simulink model "MPC_mobile_base_ROS"  (R2018b)
settings: Solver=ode4  StartTime=0.0  StopTime=inf  FixedStep=T  RelTol=1e-3
values from neighbouring files (symbols this model uses):
  N = 3    [MPC_dyn_N=3arc traj.mat]    (also in MPC_dyn_N=3arc traj_active.mat; MPC_dyn_N=3complex traj.mat; MPC_dyn_N=3complex traj_active.mat; MPC_dyn_N=6arc traj.mat = 6)
  T = 0.5    [MPC_dyn_N=3arc traj.mat]    (also in MPC_dyn_N=3arc traj_active.mat; MPC_dyn_N=3complex traj.mat; MPC_dyn_N=3complex traj_active.mat; MPC_dyn_N=6arc traj.mat)
  xd = [0 0 0 0 0 0.000654498469498 0.0758636207458 4.96526307585e-05 0.00261799387799 0.227590374774 0.000446873251435 0.00589048622548 ... (153 elements, 3x51)]    [MPC_dyn_N=3arc traj.mat]    (also in MPC_dyn_N=3arc traj_active.mat; MPC_dyn_N=3complex traj.mat = [0 0 0 0.25 0 0 0.5 0 2.44929359829e-17 0.75 -0.024302237621; MPC_dyn_N=3complex traj_active.mat = [0 0 0 0.25 0 0 0.5 0 2.44929359829e-17 0.75 -0.024302237621; MPC_dyn_N=6arc traj.mat)
undefined symbols (not defined in the file or in its folder): Angular, Linear
libraries: simulink x6, robotlib x4, sharedtransform x1
settings Model: EnablePacing=on  Creator=RaffaelePC  LastModifiedBy=francesco
settings DebuggingCC: UnderSpecifiedDimensionMsg=warning

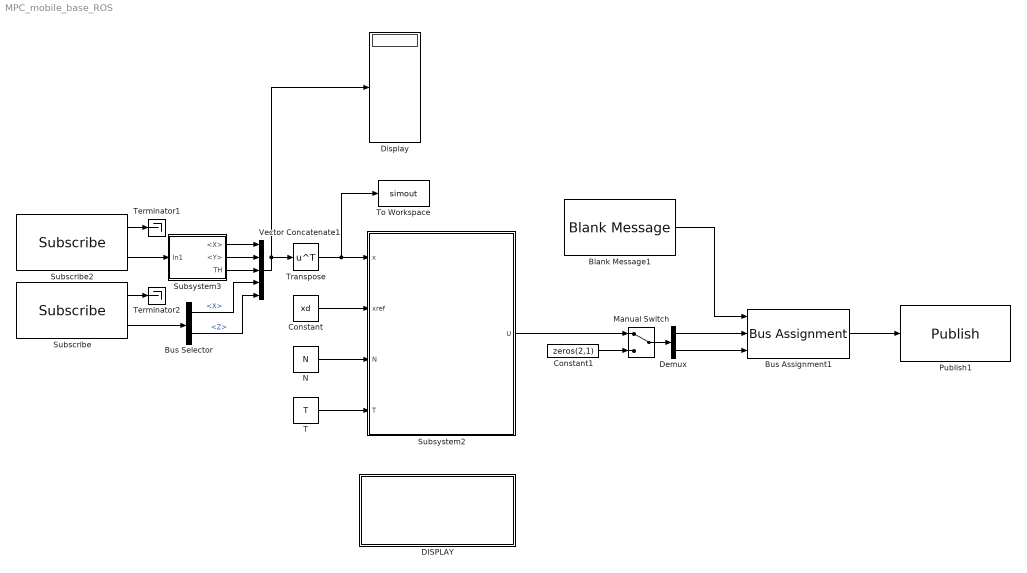
== system MPC_mobile_base_ROS ==
  Blank Message1 : robotlib/Blank Message  messageClass=Message  entityType=geometry_msgs/Twist  messageType=geometry_msgs/Twist  SampleTime=T
      settings: SourceProductBaseCode=RO
  Bus Assignment1 : BusAssignment  AssignedSignals=Linear.X,Angular.Z
  Bus Selector : BusSelector  OutputSignals=Linear.X,Angular.Z
  Constant : Constant  Value=xd
  Constant1 : Constant  Value=zeros(2,1)
  DISPLAY : Subsystem
  Demux : Demux  Outputs=2
  Display : Display
  Manual Switch : ManualSwitch
  N : Constant  Value=N
  Publish1 : robotlib/Publish  topicSource=Select from ROS network  topic=/cmd_vel  messageType=geometry_msgs/Twist  messageQueueLength=1
      settings: SourceProductBaseCode=RO
  Subscribe : robotlib/Subscribe  topicSource=Select from ROS network  topic=/cmd_vel  messageType=geometry_msgs/Twist  sampleTime=-1  messageQueueLength=1
      settings: SourceProductBaseCode=RO
  Subscribe2 : robotlib/Subscribe  topicSource=Select from ROS network  topic=/odom  messageType=nav_msgs/Odometry  sampleTime=T  messageQueueLength=1
      settings: SourceProductBaseCode=RO
  Subsystem2 : Subsystem
      mask Display: disp('MPC FINTO')
  Subsystem3 : Subsystem
  T : Constant  Value=T
  Terminator1 : Terminator
  Terminator2 : Terminator
  To Workspace : ToWorkspace  VariableName=simout  SaveFormat=Timeseries  SampleTime=-1
  Transpose : Math  Operator=transpose  SaturateOnIntegerOverflow=on
  Vector Concatenate1 : Concatenate  NumInputs=5
  wires:
  Demux/2 -> Bus Assignment1/3
  Manual Switch/1 -> Demux/1
  Constant1/1 -> Manual Switch/2
  Demux/1 -> Bus Assignment1/2
  Bus Assignment1/1 -> Publish1/1
  Blank Message1/1 -> Bus Assignment1/1
  Vector Concatenate1/1 -> Display/1, Transpose/1
  Transpose/1 -> To Workspace/1, Subsystem2/1(x)
  Constant/1 -> Subsystem2/2(xref)
  N/1 -> Subsystem2/3(N)
  T/1 -> Subsystem2/4(T)
  Subsystem2/1(U) -> Manual Switch/1
  Subsystem3/1(<X>) -> Vector Concatenate1/1
  Subsystem3/2(<Y>) -> Vector Concatenate1/2
  Subsystem3/3(TH) -> Vector Concatenate1/3
  Subscribe2/2 -> Subsystem3/1(In1)
  Subscribe2/1 -> Terminator1/1
  Subscribe/2 -> Bus Selector/1
  Bus Selector/1 -> Vector Concatenate1/4  "<X>"
  Bus Selector/2 -> Vector Concatenate1/5  "<Z>"
  Subscribe/1 -> Terminator2/1

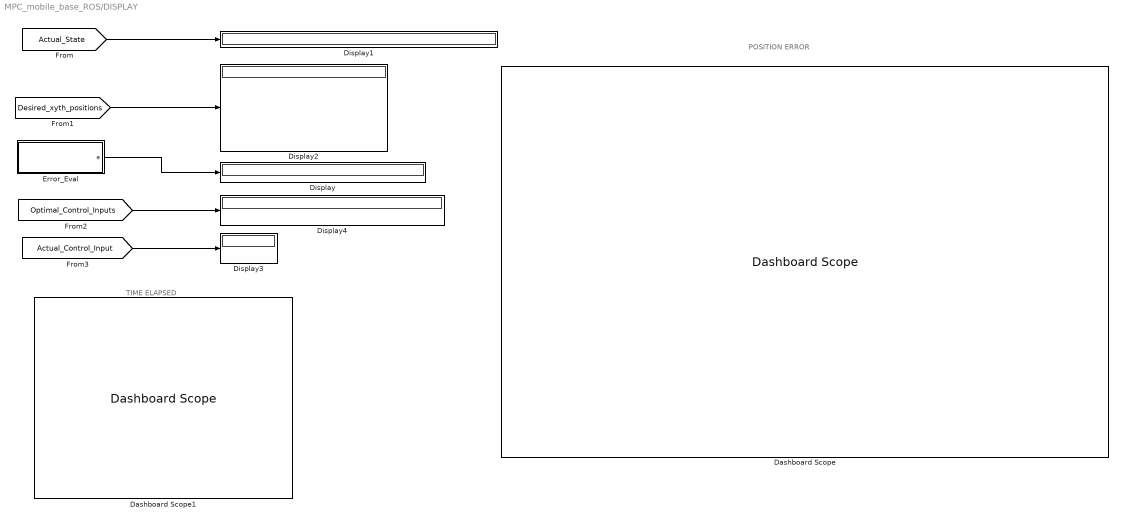
== system MPC_mobile_base_ROS/DISPLAY ==
  note: POSITION ERROR
  note: TIME ELAPSED
  Dashboard Scope : DashboardScope  WebBlockId=507  Ymin=-0.5  Ymax=0.5
  Dashboard Scope1 : DashboardScope  WebBlockId=516  Ymin=0  Ymax=1
  Display{,1..4} (5 alike) : Display
  "Error_Eval " : Subsystem
  wires:
  [Optimal_Control_Inputs] -> Display4/1
  [Desired_xyth_positions] -> Display2/1
  [Actual_Control_Input] -> Display3/1
  [Actual_State] -> Display1/1
  "Error_Eval "/1(e) -> Display/1

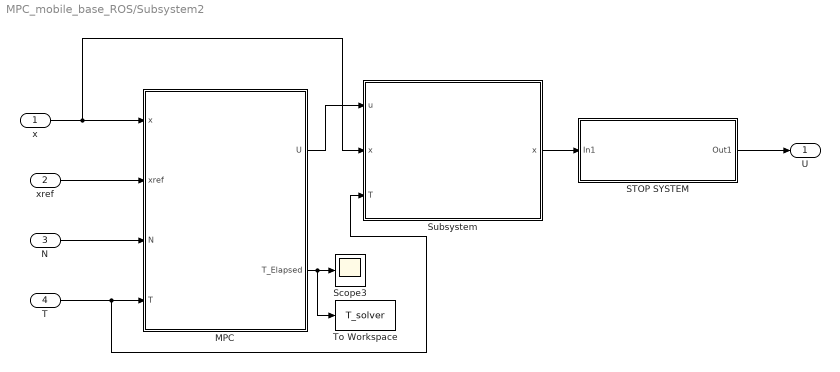
== system MPC_mobile_base_ROS/Subsystem2 ==
  x : Inport
  xref : Inport  Port=2
  N : Inport  Port=3
  T : Inport  Port=4
  MPC : Subsystem
      mask Display: fprintf('MPC CONTROLLER')
  STOP SYSTEM : Subsystem
  Scope3 : Scope
  Subsystem : Subsystem
      mask Display: disp('{\bf\fontsize{10}DYNAMIC SYSTEM}', 'texmode','on');
  To Workspace : ToWorkspace  VariableName=T_solver  SampleTime=-1
  U : Outport
  wires:
  MPC/2(T_Elapsed) -> To Workspace/1, Scope3/1
  T/1 -> Subsystem/3(T), MPC/4(T)
  N/1 -> MPC/3(N)
  xref/1 -> MPC/2(xref)
  Subsystem/1(x) -> STOP SYSTEM/1(In1)
  x/1 -> Subsystem/2("x "), MPC/1(x)
  MPC/1(U) -> Subsystem/1(u)
  STOP SYSTEM/1(Out1) -> U/1

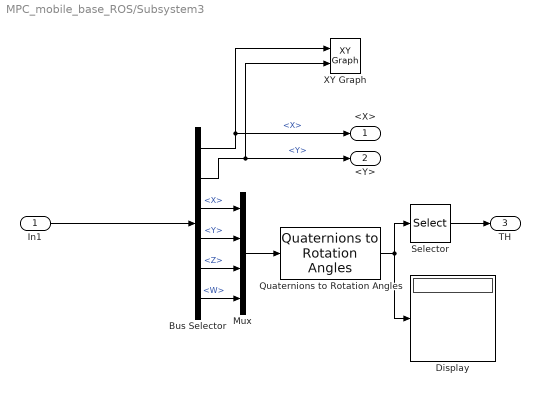
== system MPC_mobile_base_ROS/Subsystem3 ==
  In1 : Inport
  Bus Selector : BusSelector  OutputSignals=Pose.Pose.Position.X,Pose.Pose.Position.Y,Pose.Pose.Orientation.X,Pose.Pose.Orientation.Y,Pose.Pose.Orientation.Z,Pose.Pose.Orientation.W
  Display : Display
  Mux : Mux
  Quaternions to Rotation Angles : sharedtransform/Quaternions to Rotation Angles  rotationOrder=ZYX  aMode=aMode
      settings: SourceProductBaseCode=AE
  Selector : Selector  InputPortWidth=3  IndexOptions=Index vector (dialog)  Indices=3  OutputSizes=1
  XY Graph : simulink/Sinks/XY Graph  xmin=-1  xmax=10  ymin=-1  ymax=4  st=-1
  <X> : Outport
  <Y> : Outport  Port=2
  TH : Outport  Port=3
  wires:
  Bus Selector/1 -> XY Graph/1, <X>/1  "<X>"
  In1/1 -> Bus Selector/1
  Bus Selector/2 -> XY Graph/2, <Y>/1  "<Y>"
  Bus Selector/6 -> Mux/4  "<W>"
  Bus Selector/5 -> Mux/3  "<Z>"
  Bus Selector/4 -> Mux/2  "<Y>"
  Bus Selector/3 -> Mux/1  "<X>"
  Mux/1 -> Quaternions to Rotation Angles/1
  Quaternions to Rotation Angles/1 -> Selector/1, Display/1
  Selector/1 -> TH/1

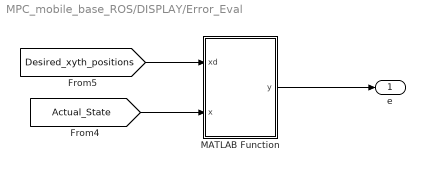
== system MPC_mobile_base_ROS/DISPLAY/Error_Eval  ==
  MATLAB Function : MATLAB Function  TreatAsAtomicUnit=on
  e : Outport
  wires:
  MATLAB Function/1(y) -> e/1
  [Desired_xyth_positions] -> MATLAB Function/1(xd)
  [Actual_State] -> MATLAB Function/2(x)

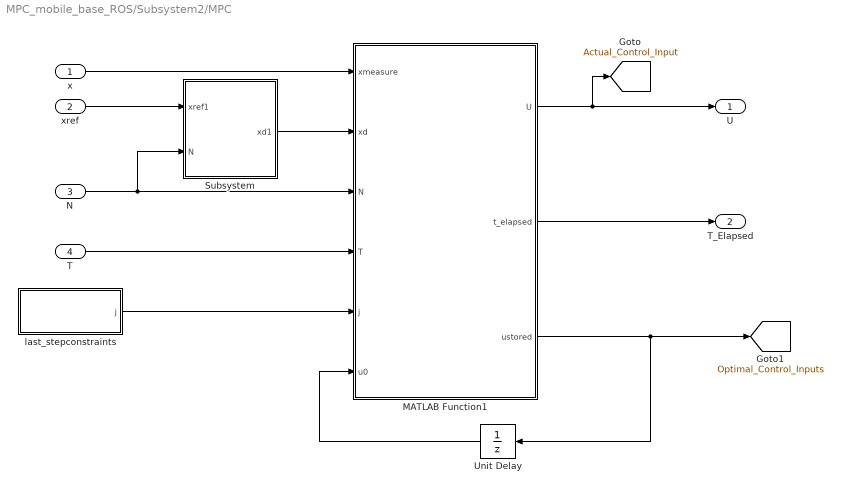
== system MPC_mobile_base_ROS/Subsystem2/MPC ==
  x : Inport
  xref : Inport  Port=2
  N : Inport  Port=3
  T : Inport  Port=4
  MATLAB Function1 : MATLAB Function  TreatAsAtomicUnit=on
  Subsystem : Subsystem
  Unit Delay : UnitDelay  InitialCondition=zeros(2,N)  SampleTime=-1
  last_stepconstraints : Subsystem
  U : Outport
  T_Elapsed : Outport  Port=2
  tag scope: Actual_Control_Input=global, Optimal_Control_Inputs=global
  wires:
  Subsystem/1(xd1) -> MATLAB Function1/2(xd)
  MATLAB Function1/1(U) -> [Actual_Control_Input], U/1
  MATLAB Function1/3(ustored) -> Unit Delay/1, [Optimal_Control_Inputs]
  Unit Delay/1 -> MATLAB Function1/6(u0)
  xref/1 -> Subsystem/1(xref1)
  x/1 -> MATLAB Function1/1(xmeasure)
  N/1 -> Subsystem/2(N), MATLAB Function1/3(N)
  T/1 -> MATLAB Function1/4(T)
  last_stepconstraints/1(j) -> MATLAB Function1/5(j)
  MATLAB Function1/2(t_elapsed) -> T_Elapsed/1

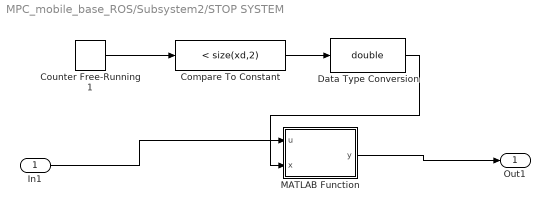
== system MPC_mobile_base_ROS/Subsystem2/STOP SYSTEM ==
  In1 : Inport
  Compare To Constant : simulink/Logic and Bit Operations/Compare To Constant  relop=<  const=size(xd,2)  OutDataTypeStr=boolean
  Counter Free-Running1 : simulink/Sources/Counter Free-Running  NumBits=12  tsamp=-1
  Data Type Conversion : DataTypeConversion  OutDataTypeStr=double
  MATLAB Function : MATLAB Function  TreatAsAtomicUnit=on
  Out1 : Outport
  wires:
  In1/1 -> MATLAB Function/1(u)
  MATLAB Function/1(y) -> Out1/1
  Counter Free-Running1/1 -> Compare To Constant/1
  Data Type Conversion/1 -> MATLAB Function/2(x)
  Compare To Constant/1 -> Data Type Conversion/1

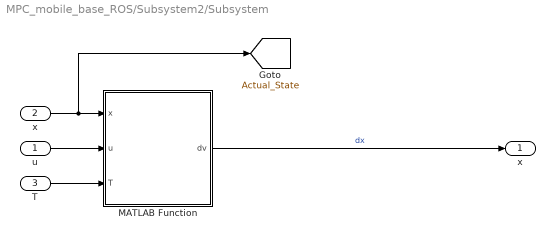
== system MPC_mobile_base_ROS/Subsystem2/Subsystem ==
  u : Inport
  "x " : Inport  Port=2
  T : Inport  Port=3
  MATLAB Function : MATLAB Function  TreatAsAtomicUnit=on
  x : Outport
  tag scope: Actual_State=global
  wires:
  u/1 -> MATLAB Function/2(u)
  MATLAB Function/1(dv) -> x/1  "dx"
  "x "/1 -> MATLAB Function/1(x), [Actual_State]
  T/1 -> MATLAB Function/3(T)

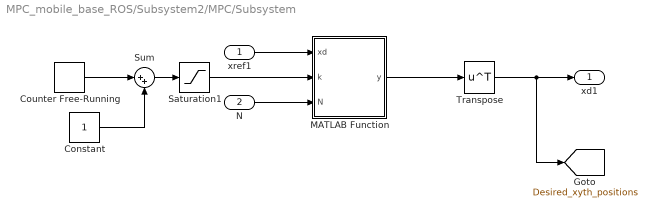
== system MPC_mobile_base_ROS/Subsystem2/MPC/Subsystem ==
  xref1 : Inport
  N : Inport  Port=2
  Constant : Constant
  Counter Free-Running : simulink/Sources/Counter Free-Running  NumBits=12  tsamp=-1
  MATLAB Function : MATLAB Function  TreatAsAtomicUnit=on
  Saturation1 : Saturate  UpperLimit=size(xd,2)
  Sum : Sum  Inputs=|++
  Transpose : Math  Operator=transpose  SaturateOnIntegerOverflow=on
  xd1 : Outport
  tag scope: Desired_xyth_positions=global
  wires:
  Transpose/1 -> [Desired_xyth_positions], xd1/1
  MATLAB Function/1(y) -> Transpose/1
  N/1 -> MATLAB Function/3(N)
  xref1/1 -> MATLAB Function/1(xd)
  Constant/1 -> Sum/2
  Counter Free-Running/1 -> Sum/1
  Sum/1 -> Saturation1/1
  Saturation1/1 -> MATLAB Function/2(k)

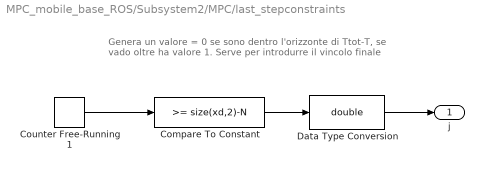
== system MPC_mobile_base_ROS/Subsystem2/MPC/last_stepconstraints ==
  note: Genera un valore = 0 se sono dentro l'orizzonte di Ttot-T, se vado oltre ha valore 1. Serve per introdurre il vincolo finale
  Compare To Constant : simulink/Logic and Bit Operations/Compare To Constant  relop=>=  const=size(xd,2)-N  OutDataTypeStr=boolean
  Counter Free-Running1 : simulink/Sources/Counter Free-Running  NumBits=12  tsamp=-1
  Data Type Conversion : DataTypeConversion  OutDataTypeStr=double
  j : Outport
  wires:
  Compare To Constant/1 -> Data Type Conversion/1
  Counter Free-Running1/1 -> Compare To Constant/1
  Data Type Conversion/1 -> j/1

== matlab function MPC_mobile_base_ROS/Subsystem2/STOP SYSTEM/MATLAB Function ==
  settings: updateMethod=DISCRETE  sampleTime=T
  data: u input; y output; x input
function y = fcn(u,x)

y = u.*x;

== matlab function MPC_mobile_base_ROS/Subsystem2/MPC/Subsystem/MATLAB Function ==
  settings: updateMethod=DISCRETE  sampleTime=T
  data: xd input; y output size=[3 N+1]; k input; N input
function y  = fcn(xd,k,N)

if size(xd,2)-k>=N
h=xd(:,k:k+N);
y=h;
else
h=[xd(:,k:end) xd(:,end)*ones(1,N-(size(xd,2)-k))];
y = h;
end

== matlab function MPC_mobile_base_ROS/Subsystem2/MPC/MATLAB Function1 ==
  settings: updateMethod=DISCRETE  sampleTime=T
  data: xmeasure input size=5; U output size=[2 1]; t_elapsed output double size=[1]; xd input; N input; T input; j input; u0 input size=[2 N]; ustored output double size=[2 N] [..20]
function [U,t_elapsed,ustored] = MPC(xmeasure,xd,N,T,j,u0)
coder.extrinsic('tic')
coder.extrinsic('toc')
coder.extrinsic('MPCSOLVER');

t_elapsed=0;

t_start=tic;

U=zeros(2,1); u = zeros(2,N);
xs=xd;
    
u0 = [u0(:,2:size(u0,2)) u0(:,size(u0,2))];

    %% dati solutore


% options = optimset('Display','off',...
%                 'TolFun', 1e-6,...
%                 'MaxIter', 10000,...
%                 'Algorithm', 'active-set',...
%                 'FinDiffType', 'forward',...
%                 'RelLineSrchBnd', [],...
%                 'RelLineSrchBndDuration', 1,...
%                 'TolConSQP', 1e-6);

%% MPC ALGORITHM 

x0=xmeasure';
t0 =0;

if size(xd,1)<N
    U=u0(:,1);
    ustored=u0(:,1:end);
    
else
    
   

    [u_new, V] = MPCSOLVER(N, t0, x0, u0, T, xs, xd,j);

%   [u_new, V] = solveOptimalControlProblem ...
%         (@runningcosts, @terminalcosts, @constraints, @terminalconstraints, ...
%         @linearconstraints, @system, N, t0, x0, u0, T, xs, xd);
     
    ustored=u_new;

    U(1)=u_new(1,1);
    U(2)=u_new(2,1);
    
    
t_elapsed=toc(t_start);

end 

end

== matlab function MPC_mobile_base_ROS/DISPLAY/Error_Eval /MATLAB Function ==
  settings: updateMethod=DISCRETE  sampleTime=T
  data: xd input; y output size=[3 1]; x input
function y = fcn(xd,x)

h = [xd(1,1)-x(1);xd(1,2)-x(2);xd(1,3)-x(3)];
y=h;

== matlab function MPC_mobile_base_ROS/Subsystem2/Subsystem/MATLAB Function ==
  settings: updateMethod=DISCRETE  sampleTime=T
  data: x input; dv output size=[2 1]; u input size=[2 1]; T input
function dv = sys_dynamics(x,u,T)

[A,F,D] = matriceseval(x.');
%       
% G=[cos(x(3)) 0  ; ...
%    sin(x(3)) 0  ; ...
%       0      1  ];

 dx=A*x.' + F*u + D;
 
 dv=x(4:5).'+dx(4:5)*T;

end
